simulink model "Full_Motor_Sim"  (R2020b)
settings: Solver=VariableStepAuto  StartTime=0.0  StopTime=1  RelTol=1e-3
libraries: fl_lib x26, ee_lib x20, nesl_utility x19, simulink x12
(part 1 of 2)
settings Model: Creator=1  LastModifiedBy=1
settings SimscapeCC: SimscapeLogType=all  SimscapeLogOpenViewer=on  SimscapeLogName=simlog_ee_igbt  SimscapeLogLimitData=off

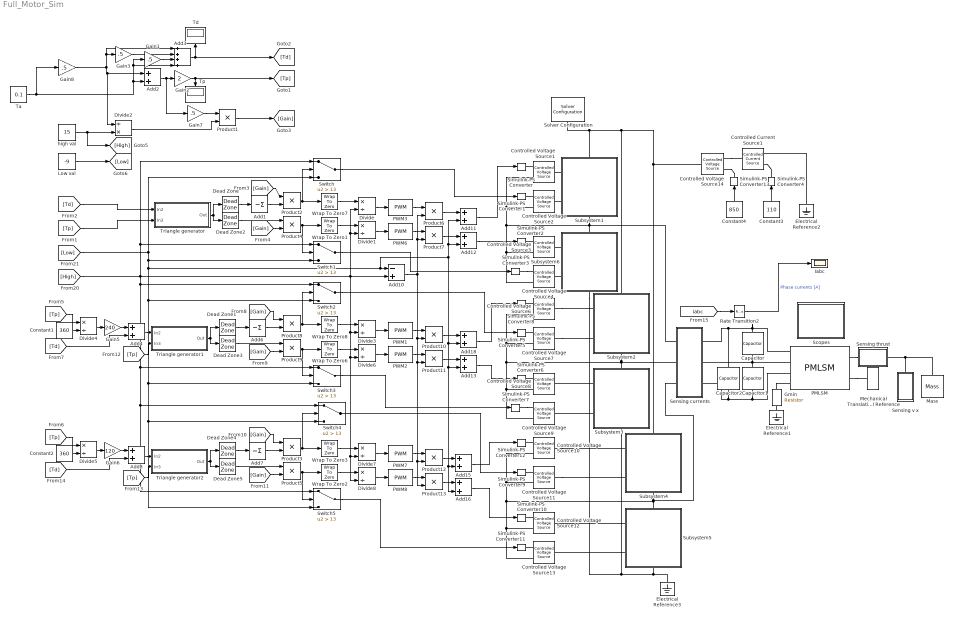
== system Full_Motor_Sim ==
  Add1 : Sum  Inputs=-
  Add10 : Sum  Inputs=-+
  Add{2,4,8,11..13,15..16,18} (9 alike) : Sum
  Add3 : Sum  Inputs=++++
  Add6 : Sum  Inputs=-
  Add7 : Sum  Inputs=-
  Capacitor : fl_lib/Electrical/Electrical Elements/Capacitor  c=1e-4 F  r=0 Ohm  g=0 1/Ohm  i_specify=off  i_priority=None  i=0 A  i_nominal_specify=off  i_nominal_unit=A  i_nominal_value=1  v_specify=off  v_priority=None  v=0 V  v_nominal_specify=off  v_nominal_unit=V  v_nominal_value=1  vc_specify=off  vc_priority=High  vc=0 V  vc_nominal_specify=off  vc_nominal_unit=V  vc_nominal_value=1
  Capacitor1 : fl_lib/Electrical/Electrical Elements/Capacitor  c=1e-4 F  r=0 Ohm  g=0 1/Ohm  i_specify=off  i_priority=None  i=0 A  i_nominal_specify=off  i_nominal_unit=A  i_nominal_value=1  v_specify=off  v_priority=None  v=0 V  v_nominal_specify=off  v_nominal_unit=V  v_nominal_value=1  vc_specify=off  vc_priority=High  vc=0 V  vc_nominal_specify=off  vc_nominal_unit=V  vc_nominal_value=1
  Capacitor2 : fl_lib/Electrical/Electrical Elements/Capacitor  c=1e-4 F  r=0 Ohm  g=0 1/Ohm  i_specify=off  i_priority=None  i=0 A  i_nominal_specify=off  i_nominal_unit=A  i_nominal_value=1  v_specify=off  v_priority=None  v=0 V  v_nominal_specify=off  v_nominal_unit=V  v_nominal_value=1  vc_specify=off  vc_priority=High  vc=0 V  vc_nominal_specify=off  vc_nominal_unit=V  vc_nominal_value=1
  Constant1 : Constant  Value=360
  Constant2 : Constant  Value=360
  Constant3 : Constant  Value=110
  Constant4 : Constant  Value=850
  Controlled Current Source1 : fl_lib/Electrical/Electrical Sources/Controlled Current Source
  Controlled Voltage Source{1..4,6..14} (13 alike) : fl_lib/Electrical/Electrical Sources/Controlled Voltage Source
  Dead Zone : DeadZone  LowerValue=0  UpperValue=18  SaturateOnIntegerOverflow=on
  Dead Zone1 : DeadZone  LowerValue=0  UpperValue=18  SaturateOnIntegerOverflow=on
  Dead Zone2 : DeadZone  LowerValue=-18  UpperValue=0  SaturateOnIntegerOverflow=on
  Dead Zone3 : DeadZone  LowerValue=-18  UpperValue=0  SaturateOnIntegerOverflow=on
  Dead Zone4 : DeadZone  LowerValue=0  UpperValue=18  SaturateOnIntegerOverflow=on
  Dead Zone5 : DeadZone  LowerValue=-18  UpperValue=0  SaturateOnIntegerOverflow=on
  Divide{,1,3..8} (8 alike) : Product  Inputs=*/
  Divide2 : Product  Inputs=/*
  Electrical Reference1 : fl_lib/Electrical/Electrical Elements/Electrical Reference
      settings: SourceProductName=Foundation Library
  Electrical Reference2 : fl_lib/Electrical/Electrical Elements/Electrical Reference
      settings: SourceProductName=Foundation Library
  Electrical Reference3 : fl_lib/Electrical/Electrical Elements/Electrical Reference
      settings: SourceProductName=Foundation Library
  Gain{1,3,7..8} (4 alike) : Gain  Gain=.5
  Gain2 : Gain  Gain=2
  Gain5 : Gain  Gain=240
  Gain6 : Gain  Gain=120
  Gmin : fl_lib/Electrical/Electrical Elements/Resistor  R=1e9 Ohm  i_specify=off  i_priority=High  i=0 A  i_nominal_specify=off  i_nominal_unit=A  i_nominal_value=1  v_specify=off  v_priority=High  v=0 V  v_nominal_specify=off  v_nominal_unit=V  v_nominal_value=1
      settings: SourceProductName=Foundation Library
  Iabc : Scope
  "Low val " : Constant  Value=-9
  Mass : fl_lib/Mechanical/Translational Elements/Mass  mass=7.5 kg  num_ports=foundation.enum.numPorts2.one  v_specify=off  v_priority=High  v=0 m/s  v_nominal_specify=off  v_nominal_unit=m/s  v_nominal_value=1  f_specify=off  f_priority=None  f=0 N  f_nominal_specify=off  f_nominal_unit=N  f_nominal_value=1
      settings: SourceProductName=Foundation Library
  Mechanical Translational Reference : fl_lib/Mechanical/Translational Elements/Mechanical Translational Reference
      settings: SourceProductName=Foundation Library
  PMLSM : ee_lib/Electromechanical/Permanent Magnet/PMLSM  winding_type=ee.enum.statorconnection.wye  machine_param=ee.enum.pmsm.parameterization.constant  polarPitch=16 mm  pmflux_param=ee.enum.pmfluxlin.backemfconstant  pm_flux_linkage=PM Wb  force_constant=0.18 N/A  back_emf_constant=15.75 s*V/m  stator_param=ee.enum.statorparam.LsLmMs  Ld=Ld H  Lq=Lq H  idVec=[-200, 0, 200] A  iqVec=[-200, 0, 200] A  LdMatrix=0.00019 * ones(3, 3) H  LqMatrix=0.00025 * ones(3, 3) H  PmMatrix=0.03 * ones(3, 3) Wb  kfMatrix=0.18 * ones(3, 3) N/A  keMatrix=0.18 * ones(3, 3) s*V/m  L0=L0 H  Ls=0.00077 H  Lm=-0.000077 H  Ms=0.0000385 H  Rs=0.254 Ohm  zero_sequence=ee.enum.park.zerosequence.include  M=7.5 kg  lam=0 N/(m/s)  axes_param=ee.enum.rotorangle.qaxis  i_d_specify=off  i_d_priority=None  i_d=0 A  i_d_nominal_specify=off  i_d_nominal_unit=A  i_d_nominal_value=1  i_q_specify=off  i_q_priority=None  i_q=0 A  i_q_nominal_specify=off  i_q_nominal_unit=A  i_q_nominal_value=1  force_specify=off  force_priority=None  force=0 N  force_nominal_specify=off  force_nominal_unit=N  force_nominal_value=1  linear_velocity_specify=off  linear_velocity_priority=High  linear_velocity=0 m/s  linear_velocity_nominal_specify=off  linear_velocity_nominal_unit=m/s  linear_velocity_nominal_value=1  linear_position_specify=off  linear_position_priority=High  linear_position=0 m  linear_position_nominal_specify=off  linear_position_nominal_unit=m  linear_position_nominal_value=1
      settings: SourceProductName=Electrical  InternalSimscapePortConfiguration="{\"Bottom\":[],\"Left\":[{\"id\":\"a\",\"label\":\"a\",\"type\":\"foundation.electrical.electrical\"},{\"id\":\"b\",\"label\":\"b\",\"type\":\"foundation.electrical.electrical\"},{\"id\":\"c\",\"label\":\"c\",\"type\":\"foundation.electrical.electrical\"},{\"id\":\"n\",\"label\":\"n\",\"type\":\"foundation.electrical.electrical\"}],\"Right\":[{\"id\":\"R\",\"label\":\"R\",\"type\":\"foundation.mechanical.translational.translational\"},{\"id\":\"C\",\"label\":\"C\",\"type\":\"foundation.mechanical.translational.translational\"}],\"Top\":[]}"
  PWM{1..3,6..8} (6 alike) : simulink/Discontinuities/PWM  DisableCoverage=on  Period=0.005  DisallowZeroDutyCycle=off  RunAtFixedTimeIntervals=off  SampleTime=0.1
  Product{1..13} (13 alike) : Product
  Rate Transition2 : RateTransition  OutPortSampleTime=Tsc
  Scopes : Subsystem
  Sensing currents : Subsystem
      mask Display: disp('iabc')
  Sensing thrust : Subsystem
      mask Display: disp('thrust')
  Sensing v x : Subsystem
      mask Display: disp('v,x')
  Simulink-PS Converter{,1..3,5..13} (13 alike) : nesl_utility/Simulink-PS Converter  PhysicalDomain=network_engine_domain  SubClassName=ps_input  LeftPortType=input  RightPortType=output  PseudoPeriodic=off  Frequencies=[]  NoiseDistribution=none  NoiseParameters=[]  Unit=V  AffineConversion=off  FilteringAndDerivatives=provide  SimscapeFilterOrder=1  InputFilterTimeConstant=0.001  UdotUserProvided=0
  Simulink-PS Converter4 : nesl_utility/Simulink-PS Converter  PhysicalDomain=network_engine_domain  SubClassName=ps_input  LeftPortType=input  RightPortType=output  PseudoPeriodic=off  Frequencies=[]  NoiseDistribution=none  NoiseParameters=[]  Unit=A  AffineConversion=off  FilteringAndDerivatives=provide  SimscapeFilterOrder=1  InputFilterTimeConstant=0.001  UdotUserProvided=0
  Solver Configuration : nesl_utility/Solver Configuration  PhysicalDomain=network_engine_domain  SubClassName=solver  LeftPortType=input  RightPortType=generic  Tones=[]  Harmonics=[]  SimulateNoise=off  Profile=off  UseLocalSampling=off  EnableSwitchedLinearOptims=on  FrequencyDomain=off  UseCCode=off  RelTol=0.001  AbsTol=1e-06  MinStep=1e-09  ToWorkspace=off  RevertToSquareIcSolve=off  NumHomotopyIterations=100  PhasorMode=off  PhasorModeNumHarmonics=1  DoDC=on  ResidualTolerance=1e-9  UseLocalSolver=on  LocalSolverChoice=NE_BACKWARD_EULER_ADVANCER  LocalSolverSampleTime=5e-6  DoFixedCost=off  MaxNonlinIter=50  MaxModeIter=2  ComputeImpulses=on  ImpulseIterations=2  LinearAlgebra=auto  EquationFormulation=NE_TIME_EF  DelaysMemoryBudget=2048  AutomaticFiltering=on  FilteringTimeConstant=0.001  PartitionStorageMethod=AS_NEEDED  PartitionMemoryBudget=1024  PartitionMethod=FAST
      settings: SourceProductName=Utilities
  Subsystem1 : Subsystem
      settings: PortSchema="{\"entries\":[{\"content\":{\"sides\":[{\"content\":{\"connectorIds\":[\"LConn1\",\"LConn2\"]},\"type\":\"ConnectorPlacement.EquallySpacedRectSide\",\"uuid\":\"28828598-fa48-4158-b9b9-1a24f22427e6\"},{\"content\":{\"connectorIds\":[],\"side\":\"RIGHT\"},\"type\":\"ConnectorPlacement.EquallySpacedRectSide\",\"uuid\":\"019dad23-614b-4455-8161-a0bd3c38edbe\"},{\"content\":{\"connectorIds\":[\"LConn3\"],\"side\":\"TOP\"},\"type\":\"ConnectorPlacement.EquallySpacedRectSide\",\"uuid\":\"f897a393-49e1-4ff6-9d33-08f3737db00c\"},{\"content\":{\"connectorIds\":[\"RConn1\"],\"side\":\"BOTTOM\"},\"type\":\"ConnectorPlacement.EquallySpacedRectSide\",\"uuid\":\"06fb1490-05e8-4341-9bc6-3d6044d20c9b\"},{\"content\":{\"connectorIds\":[],\"side\":\"HIDDEN\"},\"type\":\"ConnectorPlacement.EquallySpacedRectSide\",\"uuid\":\"25a0668a-edb0-4932-9c2b-b08682b30f2f\"}]},\"type\":\"ConnectorPlacement.EquallySpacedConnector\",\"uuid\":\"66e20cb6-4eb1-4857-9faa-51f0324dd946\"}],\"packageUris\":[\"http://schema.mathworks.com/mf0/Connector/R2020b\"],\"version\":\"1.0\"}"
  Subsystem2 : Subsystem
      settings: PortSchema="{\"entries\":[{\"content\":{\"sides\":[{\"content\":{\"connectorIds\":[\"LConn1\",\"LConn2\"]},\"type\":\"ConnectorPlacement.EquallySpacedRectSide\",\"uuid\":\"28828598-fa48-4158-b9b9-1a24f22427e6\"},{\"content\":{\"connectorIds\":[],\"side\":\"RIGHT\"},\"type\":\"ConnectorPlacement.EquallySpacedRectSide\",\"uuid\":\"019dad23-614b-4455-8161-a0bd3c38edbe\"},{\"content\":{\"connectorIds\":[\"LConn3\"],\"side\":\"TOP\"},\"type\":\"ConnectorPlacement.EquallySpacedRectSide\",\"uuid\":\"f897a393-49e1-4ff6-9d33-08f3737db00c\"},{\"content\":{\"connectorIds\":[\"RConn1\"],\"side\":\"BOTTOM\"},\"type\":\"ConnectorPlacement.EquallySpacedRectSide\",\"uuid\":\"06fb1490-05e8-4341-9bc6-3d6044d20c9b\"},{\"content\":{\"connectorIds\":[],\"side\":\"HIDDEN\"},\"type\":\"ConnectorPlacement.EquallySpacedRectSide\",\"uuid\":\"25a0668a-edb0-4932-9c2b-b08682b30f2f\"}]},\"type\":\"ConnectorPlacement.EquallySpacedConnector\",\"uuid\":\"66e20cb6-4eb1-4857-9faa-51f0324dd946\"}],\"packageUris\":[\"http://schema.mathworks.com/mf0/Connector/R2020b\"],\"version\":\"1.0\"}"
  Subsystem3 : Subsystem
      settings: PortSchema="{\"entries\":[{\"content\":{\"sides\":[{\"content\":{\"connectorIds\":[\"LConn1\",\"LConn2\"]},\"type\":\"ConnectorPlacement.EquallySpacedRectSide\",\"uuid\":\"28828598-fa48-4158-b9b9-1a24f22427e6\"},{\"content\":{\"connectorIds\":[],\"side\":\"RIGHT\"},\"type\":\"ConnectorPlacement.EquallySpacedRectSide\",\"uuid\":\"019dad23-614b-4455-8161-a0bd3c38edbe\"},{\"content\":{\"connectorIds\":[\"LConn3\"],\"side\":\"TOP\"},\"type\":\"ConnectorPlacement.EquallySpacedRectSide\",\"uuid\":\"f897a393-49e1-4ff6-9d33-08f3737db00c\"},{\"content\":{\"connectorIds\":[\"RConn1\"],\"side\":\"BOTTOM\"},\"type\":\"ConnectorPlacement.EquallySpacedRectSide\",\"uuid\":\"e6a9b99e-6cfc-43a0-9f1a-1d6bb159a832\"},{\"content\":{\"connectorIds\":[],\"side\":\"HIDDEN\"},\"type\":\"ConnectorPlacement.EquallySpacedRectSide\",\"uuid\":\"25a0668a-edb0-4932-9c2b-b08682b30f2f\"}]},\"type\":\"ConnectorPlacement.EquallySpacedConnector\",\"uuid\":\"66e20cb6-4eb1-4857-9faa-51f0324dd946\"}],\"packageUris\":[\"http://schema.mathworks.com/mf0/Connector/R2020b\"],\"version\":\"1.0\"}"
  Subsystem4 : Subsystem
      settings: PortSchema="{\"entries\":[{\"content\":{\"sides\":[{\"content\":{\"connectorIds\":[\"LConn1\",\"LConn2\"]},\"type\":\"ConnectorPlacement.EquallySpacedRectSide\",\"uuid\":\"28828598-fa48-4158-b9b9-1a24f22427e6\"},{\"content\":{\"connectorIds\":[],\"side\":\"RIGHT\"},\"type\":\"ConnectorPlacement.EquallySpacedRectSide\",\"uuid\":\"019dad23-614b-4455-8161-a0bd3c38edbe\"},{\"content\":{\"connectorIds\":[\"LConn3\"],\"side\":\"TOP\"},\"type\":\"ConnectorPlacement.EquallySpacedRectSide\",\"uuid\":\"f897a393-49e1-4ff6-9d33-08f3737db00c\"},{\"content\":{\"connectorIds\":[\"RConn1\"],\"side\":\"BOTTOM\"},\"type\":\"ConnectorPlacement.EquallySpacedRectSide\",\"uuid\":\"06fb1490-05e8-4341-9bc6-3d6044d20c9b\"},{\"content\":{\"connectorIds\":[],\"side\":\"HIDDEN\"},\"type\":\"ConnectorPlacement.EquallySpacedRectSide\",\"uuid\":\"25a0668a-edb0-4932-9c2b-b08682b30f2f\"}]},\"type\":\"ConnectorPlacement.EquallySpacedConnector\",\"uuid\":\"66e20cb6-4eb1-4857-9faa-51f0324dd946\"}],\"packageUris\":[\"http://schema.mathworks.com/mf0/Connector/R2020b\"],\"version\":\"1.0\"}"
  Subsystem5 : Subsystem
      settings: PortSchema="{\"entries\":[{\"content\":{\"sides\":[{\"content\":{\"connectorIds\":[\"LConn1\",\"LConn2\"]},\"type\":\"ConnectorPlacement.EquallySpacedRectSide\",\"uuid\":\"28828598-fa48-4158-b9b9-1a24f22427e6\"},{\"content\":{\"connectorIds\":[],\"side\":\"RIGHT\"},\"type\":\"ConnectorPlacement.EquallySpacedRectSide\",\"uuid\":\"019dad23-614b-4455-8161-a0bd3c38edbe\"},{\"content\":{\"connectorIds\":[\"LConn3\"],\"side\":\"TOP\"},\"type\":\"ConnectorPlacement.EquallySpacedRectSide\",\"uuid\":\"f897a393-49e1-4ff6-9d33-08f3737db00c\"},{\"content\":{\"connectorIds\":[\"RConn1\"],\"side\":\"BOTTOM\"},\"type\":\"ConnectorPlacement.EquallySpacedRectSide\",\"uuid\":\"e6a9b99e-6cfc-43a0-9f1a-1d6bb159a832\"},{\"content\":{\"connectorIds\":[],\"side\":\"HIDDEN\"},\"type\":\"ConnectorPlacement.EquallySpacedRectSide\",\"uuid\":\"25a0668a-edb0-4932-9c2b-b08682b30f2f\"}]},\"type\":\"ConnectorPlacement.EquallySpacedConnector\",\"uuid\":\"66e20cb6-4eb1-4857-9faa-51f0324dd946\"}],\"packageUris\":[\"http://schema.mathworks.com/mf0/Connector/R2020b\"],\"version\":\"1.0\"}"
  Subsystem6 : Subsystem
      settings: PortSchema="{\"entries\":[{\"content\":{\"sides\":[{\"content\":{\"connectorIds\":[\"LConn1\",\"LConn2\"]},\"type\":\"ConnectorPlacement.EquallySpacedRectSide\",\"uuid\":\"28828598-fa48-4158-b9b9-1a24f22427e6\"},{\"content\":{\"connectorIds\":[],\"side\":\"RIGHT\"},\"type\":\"ConnectorPlacement.EquallySpacedRectSide\",\"uuid\":\"019dad23-614b-4455-8161-a0bd3c38edbe\"},{\"content\":{\"connectorIds\":[\"LConn3\"],\"side\":\"TOP\"},\"type\":\"ConnectorPlacement.EquallySpacedRectSide\",\"uuid\":\"f897a393-49e1-4ff6-9d33-08f3737db00c\"},{\"content\":{\"connectorIds\":[\"RConn1\"],\"side\":\"BOTTOM\"},\"type\":\"ConnectorPlacement.EquallySpacedRectSide\",\"uuid\":\"e6a9b99e-6cfc-43a0-9f1a-1d6bb159a832\"},{\"content\":{\"connectorIds\":[],\"side\":\"HIDDEN\"},\"type\":\"ConnectorPlacement.EquallySpacedRectSide\",\"uuid\":\"25a0668a-edb0-4932-9c2b-b08682b30f2f\"}]},\"type\":\"ConnectorPlacement.EquallySpacedConnector\",\"uuid\":\"66e20cb6-4eb1-4857-9faa-51f0324dd946\"}],\"packageUris\":[\"http://schema.mathworks.com/mf0/Connector/R2020b\"],\"version\":\"1.0\"}"
  Switch{,1..5} (6 alike) : Switch  Criteria=u2 > Threshold  Threshold=13
  Ta : Constant  Value=0.1
  Td : Display
  Tp : Display
  Triangle generator : Subsystem
  Triangle generator1 : Subsystem
  Triangle generator2 : Subsystem
  Wrap To Zero{1..3,6..8} (6 alike) : simulink/Discontinuities/Wrap To Zero  Threshold=15
      settings: SourceProductBaseCode=SL
  "high val " : Constant  Value=15
  wires:
  Gain2/1 -> [Tp], Tp/1
  [Tp] -> Triangle generator/2(In3)
  Ta/1 -> Gain8/1, Gain1/1, Add3/4, Add2/2
  Add2/1 -> Gain7/1, Gain2/1
  Gain8/1 -> Add2/1, Divide2/1, Gain3/1, Add3/1
  Dead Zone/1 -> Add1/1
  Triangle generator/1(Out) -> Dead Zone/1, Dead Zone2/1
  Gain1/1 -> Add3/3
  [Td] -> Triangle generator/1(In2)
  Add1/1 -> Product2/2
  [Gain] -> Product2/1
  Dead Zone2/1 -> Product4/1
  [Gain] -> Product4/2
  [Tp] -> Divide4/1
  Constant1/1 -> Divide4/2
  Divide4/1 -> Gain5/1
  Divide5/1 -> Gain6/1
  Constant2/1 -> Divide5/2
  [Tp] -> Divide5/1
  Gain5/1 -> Add4/1
  Gain6/1 -> Add8/1
  [Td] -> Add4/2
  [Gain] -> Product9/2
  Dead Zone3/1 -> Product9/1
  [Gain] -> Product8/1
  Add6/1 -> Product8/2
  Triangle generator1/1(Out) -> Dead Zone3/1, Dead Zone1/1
  Dead Zone1/1 -> Add6/1
  Add4/1 -> Triangle generator1/1(In2)
  Dead Zone4/1 -> Add7/1
  Triangle generator2/1(Out) -> Dead Zone4/1, Dead Zone5/1
  Add7/1 -> Product3/2
  [Gain] -> Product3/1
  Dead Zone5/1 -> Product5/1
  [Gain] -> Product5/2
  Add8/1 -> Triangle generator2/1(In2)
  [Tp] -> Triangle generator2/2(In3)
  [Tp] -> Triangle generator1/2(In3)
  "high val "/1 -> [High], Divide2/2
  Gain7/1 -> Product1/1
  Divide2/1 -> Product1/2
  Product1/1 -> [Gain]
  Product2/1 -> Switch/2, Wrap To Zero7/1
  Product4/1 -> Switch1/2, Wrap To Zero1/1
  [Td] -> Add8/2
  Product8/1 -> Wrap To Zero8/1, Switch2/2
  Product3/1 -> Switch4/2, Wrap To Zero3/1
  Product5/1 -> Switch5/2, Wrap To Zero2/1
  Product9/1 -> Wrap To Zero6/1, Switch3/2
  [Low] -> Switch2/3, Switch3/3, Switch4/3, Switch5/3, Add18/2, Add13/2, Add16/2, Add15/2, Add11/2, Add12/2, Add10/1, Switch1/3, Switch/3
  Switch5/1 -> Simulink-PS Converter11/1
  Switch4/1 -> Simulink-PS Converter9/1
  Switch2/1 -> Simulink-PS Converter5/1
  Switch3/1 -> Simulink-PS Converter7/1
  Switch1/1 -> Simulink-PS Converter3/1
  Wrap To Zero7/1 -> Divide/1
  Wrap To Zero1/1 -> Divide1/1
  Divide/1 -> PWM3/1
  Divide1/1 -> PWM6/1
  PWM3/1 -> Product6/1
  PWM6/1 -> Product7/1
  Add3/1 -> Td/1, [Td]
  PWM2/1 -> Product11/1
  PWM1/1 -> Product10/1
  Divide6/1 -> PWM2/1
  Divide3/1 -> PWM1/1
  Wrap To Zero6/1 -> Divide6/1
  Wrap To Zero8/1 -> Divide3/1
  Wrap To Zero3/1 -> Divide7/1
  Wrap To Zero2/1 -> Divide8/1
  [High] -> Switch3/1, Switch4/1, Switch5/1, Switch2/1, Switch1/1, Switch/1, Add10/2, Divide3/2, Divide6/2, Divide8/2, Divide7/2, Divide/2, Divide1/2
  Divide7/1 -> PWM7/1
  Divide8/1 -> PWM8/1
  PWM7/1 -> Product12/1
  PWM8/1 -> Product13/1
  Switch/1 -> Simulink-PS Converter1/1
  Add10/1 -> Product7/2, Product6/2, Product12/2, Product13/2, Product11/2, Product10/2
  "Low val "/1 -> [Low]
  Product6/1 -> Add11/1
  Product7/1 -> Add12/1
  Product11/1 -> Add13/1
  Product10/1 -> Add18/1
  Product13/1 -> Add16/1
  Product12/1 -> Add15/1
  Add11/1 -> Simulink-PS Converter/1
  Add12/1 -> Simulink-PS Converter2/1
  Add18/1 -> Simulink-PS Converter8/1
  Add13/1 -> Simulink-PS Converter6/1
  Add15/1 -> Simulink-PS Converter12/1
  Add16/1 -> Simulink-PS Converter10/1
  Constant3/1 -> Simulink-PS Converter4/1
  Gain3/1 -> Add3/2
  Constant4/1 -> Simulink-PS Converter13/1
  [iabc] -> Rate Transition2/1
  Rate Transition2/1 -> Iabc/1  "Phase currents [A]"
  connections:
  Controlled Voltage Source3/RConn2 -- Sensing currents/LConn1 -- Subsystem6/LConn3 -- Subsystem1/RConn1 -- Controlled Voltage Source2/RConn2 -- Controlled Voltage Source1/RConn2 -- Controlled Voltage Source4/RConn2
  Simulink-PS Converter/RConn1 -- Controlled Voltage Source1/RConn1
  Simulink-PS Converter1/RConn1 -- Controlled Voltage Source2/RConn1
  Simulink-PS Converter2/RConn1 -- Controlled Voltage Source3/RConn1
  Simulink-PS Converter3/RConn1 -- Controlled Voltage Source4/RConn1
  Subsystem1/LConn1 -- Controlled Voltage Source1/LConn1
  Subsystem1/LConn2 -- Controlled Voltage Source2/LConn1
  Subsystem6/LConn1 -- Controlled Voltage Source3/LConn1
  Subsystem6/LConn2 -- Controlled Voltage Source4/LConn1
  Controlled Voltage Source7/RConn2 -- Controlled Voltage Source8/RConn2 -- Controlled Voltage Source9/RConn2 -- Subsystem2/RConn1 -- Subsystem3/LConn3 -- Sensing currents/LConn2 -- Controlled Voltage Source6/RConn2
  Subsystem3/LConn1 -- Controlled Voltage Source8/LConn1
  Simulink-PS Converter7/RConn1 -- Controlled Voltage Source9/RConn1
  Capacitor/RConn1 -- PMLSM/LConn2 -- Capacitor1/LConn1 -- Sensing currents/RConn2
  Simulink-PS Converter6/RConn1 -- Controlled Voltage Source8/RConn1
  Simulink-PS Converter5/RConn1 -- Controlled Voltage Source7/RConn1
  Controlled Voltage Source7/LConn1 -- Subsystem2/LConn2
  Controlled Voltage Source6/LConn1 -- Subsystem2/LConn1
  Subsystem3/LConn2 -- Controlled Voltage Source9/LConn1
  Simulink-PS Converter8/RConn1 -- Controlled Voltage Source6/RConn1
  Subsystem4/RConn1 -- Sensing currents/LConn3 -- Subsystem5/LConn3 -- Controlled Voltage Source13/RConn2 -- Controlled Voltage Source12/RConn2 -- Controlled Voltage Source11/RConn2 -- Controlled Voltage Source10/RConn2
  Simulink-PS Converter12/RConn1 -- Controlled Voltage Source10/RConn1
  Subsystem5/LConn2 -- Controlled Voltage Source13/LConn1
  Controlled Voltage Source10/LConn1 -- Subsystem4/LConn1
  Simulink-PS Converter10/RConn1 -- Controlled Voltage Source12/RConn1
  Capacitor1/RConn1 -- PMLSM/LConn3 -- Capacitor2/RConn1 -- Sensing currents/RConn3
  Simulink-PS Converter11/RConn1 -- Controlled Voltage Source13/RConn1
  Subsystem5/LConn1 -- Controlled Voltage Source12/LConn1
  Simulink-PS Converter9/RConn1 -- Controlled Voltage Source11/RConn1
  Controlled Voltage Source11/LConn1 -- Subsystem4/LConn2
  Simulink-PS Converter4/RConn1 -- Controlled Current Source1/RConn1
  Subsystem4/LConn3 -- Controlled Voltage Source14/LConn1 -- Subsystem2/LConn3 -- Subsystem1/LConn3 -- Solver Configuration/RConn1
  Subsystem5/RConn1 -- Electrical Reference3/LConn1 -- Subsystem6/RConn1 -- Subsystem3/RConn1
  Electrical Reference2/LConn1 -- Controlled Current Source1/RConn2
  Controlled Voltage Source14/RConn2 -- Controlled Current Source1/LConn1
  Controlled Voltage Source14/RConn1 -- Simulink-PS Converter13/RConn1
  Sensing thrust/RConn1 -- Mass/LConn1 -- Sensing v x/LConn1
  Electrical Reference1/LConn1 -- Gmin/LConn1
  Capacitor/LConn1 -- PMLSM/LConn1 -- Capacitor2/LConn1 -- Sensing currents/RConn1
  PMLSM/RConn1 -- Sensing thrust/LConn1
  PMLSM/RConn2 -- Mechanical Translational Reference/LConn1
  PMLSM/LConn4 -- Gmin/RConn1

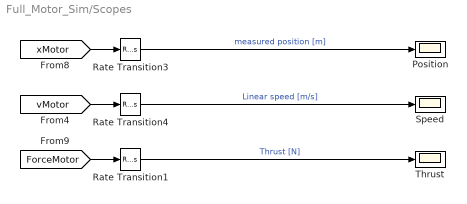
== system Full_Motor_Sim/Scopes ==
  Position : Scope
  Rate Transition1 : RateTransition  OutPortSampleTime=Tsc
  Rate Transition3 : RateTransition  OutPortSampleTime=Tsc
  Rate Transition4 : RateTransition  OutPortSampleTime=Tsc
  Speed : Scope
  Thrust : Scope
  wires:
  Rate Transition4/1 -> Speed/1  "Linear speed [m/s]"
  Rate Transition3/1 -> Position/1  "measured position [m]"
  [xMotor] -> Rate Transition3/1
  Rate Transition1/1 -> Thrust/1  "Thrust [N]"
  [ForceMotor] -> Rate Transition1/1
  [vMotor] -> Rate Transition4/1

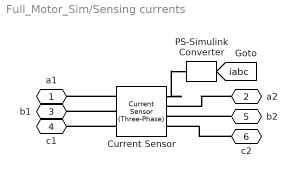
== system Full_Motor_Sim/Sensing currents ==
  Current Sensor : ee_lib/Sensors & Transducers/Current Sensor (Three-Phase)
      settings: SourceProductName=Electrical  InternalSimscapePortConfiguration="{\"Bottom\":[],\"Left\":[{\"id\":\"a1\",\"label\":\"a1\",\"type\":\"foundation.electrical.electrical\"},{\"id\":\"b1\",\"label\":\"b1\",\"type\":\"foundation.electrical.electrical\"},{\"id\":\"c1\",\"label\":\"c1\",\"type\":\"foundation.electrical.electrical\"}],\"Right\":[{\"id\":\"I_output\",\"label\":\"I\",\"type\":\"output\"},{\"id\":\"a2\",\"label\":\"a2\",\"type\":\"foundation.electrical.electrical\"},{\"id\":\"b2\",\"label\":\"b2\",\"type\":\"foundation.electrical.electrical\"},{\"id\":\"c2\",\"label\":\"c2\",\"type\":\"foundation.electrical.electrical\"}],\"Top\":[]}"
  PS-Simulink Converter : nesl_utility/PS-Simulink Converter  PhysicalDomain=network_engine_domain  SubClassName=ps_output  LeftPortType=input  RightPortType=output  PseudoPeriodic=off  Frequencies=[]  Unit=A  AffineConversion=off
      settings: SourceProductName=Utilities
  a1 : PMIOPort  Side=Left
  a2 : PMIOPort  Port=2  Side=Right
  b1 : PMIOPort  Port=3  Side=Left
  c1 : PMIOPort  Port=4  Side=Left
  b2 : PMIOPort  Port=5  Side=Right
  c2 : PMIOPort  Port=6  Side=Right
  tag scope: iabc=global
  wires:
  PS-Simulink Converter/1 -> [iabc]
  connections:
  Current Sensor/LConn1 -- a1/RConn1
  a2/RConn1 -- Current Sensor/RConn2
  Current Sensor/RConn1 -- PS-Simulink Converter/LConn1
  Current Sensor/LConn2 -- b1/RConn1
  Current Sensor/LConn3 -- c1/RConn1
  b2/RConn1 -- Current Sensor/RConn3
  c2/RConn1 -- Current Sensor/RConn4

== system Full_Motor_Sim/Sensing thrust ==
  Ideal Force Sensor : fl_lib/Mechanical/Mechanical Sensors/Ideal Force Sensor
      settings: SourceProductName=Foundation Library
  PS-Simulink Converter2 : nesl_utility/PS-Simulink Converter  PhysicalDomain=network_engine_domain  SubClassName=ps_output  LeftPortType=input  RightPortType=output  PseudoPeriodic=off  Frequencies=[]  Unit=N  AffineConversion=off
      settings: SourceProductName=Utilities
  C : PMIOPort  Side=Right
  R : PMIOPort  Port=2  Side=Left
  tag scope: ForceMotor=global
  wires:
  PS-Simulink Converter2/1 -> [ForceMotor]
  connections:
  Ideal Force Sensor/RConn1 -- C/RConn1
  Ideal Force Sensor/RConn2 -- PS-Simulink Converter2/LConn1
  Ideal Force Sensor/LConn1 -- R/RConn1

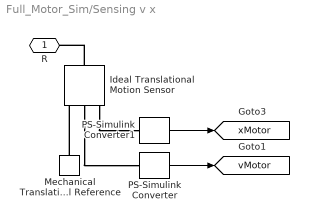
== system Full_Motor_Sim/Sensing v x ==
  Ideal Translational Motion Sensor : fl_lib/Mechanical/Mechanical Sensors/Ideal Translational Motion Sensor  offset=0 m
      settings: SourceProductName=Foundation Library
  Mechanical Translational Reference : fl_lib/Mechanical/Translational Elements/Mechanical Translational Reference
      settings: SourceProductName=Foundation Library
  PS-Simulink Converter : nesl_utility/PS-Simulink Converter  PhysicalDomain=network_engine_domain  SubClassName=ps_output  LeftPortType=input  RightPortType=output  PseudoPeriodic=off  Frequencies=[]  Unit=m/s  AffineConversion=off
      settings: SourceProductName=Utilities
  PS-Simulink Converter1 : nesl_utility/PS-Simulink Converter  PhysicalDomain=network_engine_domain  SubClassName=ps_output  LeftPortType=input  RightPortType=output  PseudoPeriodic=off  Frequencies=[]  Unit=m  AffineConversion=off
      settings: SourceProductName=Utilities
  R : PMIOPort  Side=Left
  tag scope: vMotor=global, xMotor=global
  wires:
  PS-Simulink Converter1/1 -> [xMotor]
  PS-Simulink Converter/1 -> [vMotor]
  connections:
  Ideal Translational Motion Sensor/RConn2 -- PS-Simulink Converter/LConn1
  Ideal Translational Motion Sensor/LConn1 -- R/RConn1
  Ideal Translational Motion Sensor/RConn3 -- PS-Simulink Converter1/LConn1
  Mechanical Translational Reference/LConn1 -- Ideal Translational Motion Sensor/RConn1

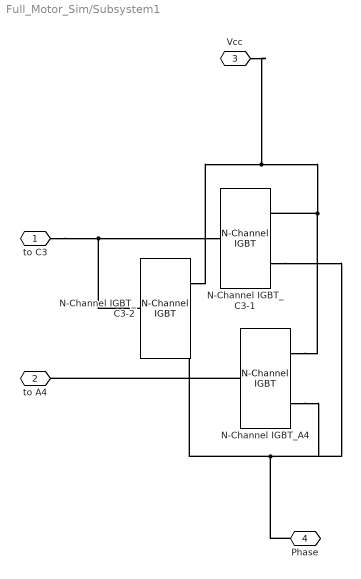
== system Full_Motor_Sim/Subsystem1 ==
  N-Channel IGBT_A4 : ee_lib/Semiconductors & Converters/N-Channel IGBT  model_type=1  Ices=25 uA  Vces=1200 V  Vth=5 V  Vce_sat=1.4 V  Ice_sat=110 A  Vge_sat=15 V  ec=1.3  Tmeas=25 degC  Vge_vec=[ -2 6 7 8 10 12 15 20 ] V  Vce_vec=[ -1 0 0.5 1 1.5 2 2.5 3 3.5 4 ] V  T_vec=[25, 125] degC  Ic_mat=[ -1.015e-5 1.35e-8 4.7135e-4 5.092e-4 5.105e-4 5.117500000000001e-4 5.1299e-4 5.1423e-4 5.1548e-4 5.1672e-4; -9.986899999999999e-6 1.35e-8 4.7135e-4 5.092e-4 5.105e-4 5.117500000000001e-4 5.1299e-4 5.1423e-4 5.1548e-4 5.1672e-4; -9.955e-6 1.35e-8 0.0065225 3.3324 48.154 93.661 105.52 105.72 105.93 106.14; -9.955e-6 1.35e-8 0.0065235 3.5783 70.264 166.33 252.4 317.67 353.38 357.39; -9.955e-6 1.35e-8 0.006524 3.7206 89.17100000000001 228.09 371.63 511.02 642.6900000000001 764.04; -9.9549e-6 1.35e-8 0.0065242 3.7716 97.79300000000001 256.21 424.27 592.92 759.2 921.52; -9.9549e-6 1.35e-8 0.0065243 3.8067 104.52 278.11 464.6 654.37 844.5700000000001 1.0339e+3; -9.9549e-6 1.35e-8 0.0065244 3.8324 109.92 295.67 496.54 702.28 909.96 1.1183e+3 ] A  Ic_mat_3D=zeros(8, 10, 2) A  C_param=3  C_GE=23.7 nF  C_GC=2.7 nF  C_CE=0 nF  C_ies=9.85 nF  C_res=218 pF  C_oes=580 pF  C_GE_vec=[ 25 31 26.5 24.9 25 24.9 24.6 24.7 24.8 ] nF  C_GC_vec=[ 55 9 5.5 3.1 2.5 2.1 1.9 1.8 1.7 ] nF  C_CE_vec=[ 5 11 6.5 4.9 3.5 2.7 2.1 1.7 1.4 ] nF  C_ies_vec=[70 62 60 60 60 60 60 60 60 ] nF  C_res_vec=[ 12 0.46 0.32 0.28 0.24 0.22 0.2 0.19 0.16 ] nF  C_oes_vec=[ 31 0.73 0.515 0.44 0.38 0.34 0.31 0.29 0.28 ] nF  C_Vce_vec=[ 0 5 10 15 20 25 30 35 40 ] V  charge_linearity_param=1  C_OX=20 nF  V_C_OX=-5 V  TF=0 ns  VAF=350 V  RC=0.0001 Ohm  RE=0.0045 Ohm  RG=1 Ohm  BF=100  T_param=2  Ices_T2=620 uA  EG=0.0001 eV  Vce_sat_T2=1.6 V  Tmeas2=150 degC  XTI=1  BEX=-0.6  RG_alpha=1 1/K  Tdevice=150 degC  Tdevice_3D=25 degC  thermal_network_parameterization=ee.enum.thermalNetworkTopology.cauer  Rth=[0, 10] K/W  Rth_Foster=[4, 6] K/W  thermal_mass_parameterization=ee.enum.thermalNetwork.timeconstant  thermal_mass=[0, 1] J/K  thermal_mass_Foster=[1.5, 3] J/K  thermal_time_constant=[0, 10] s  thermal_time_constant_Foster=[6, 18] s  thermal_mass_initial_temperatures=[25, 25] degC  Ic_vec1=[0, 10, 50, 100, 200, 400, 600] A  Vce_vec1=[0, 1.1, 1.3, 1.45, 1.75, 2.25, 2.7] V  Rmiller=0.1 Ohm  Goff=1e-5 1/Ohm  t_on=0.07 us  t_rise=0.7 us  t_off=0.2 us  t_fall=0.5 us  v_meas=300 V  Tj_vec1=[298.15, 398.15] K  Vce_mat1=[0, 1.1, 1.3, 1.45, 1.75, 2.25, 2.7; 0, 1, 1.15, 1.35, 1.7, 2.35, 3] V  E_turn_on_mat1=[0, .2, 1, 2, 4, 8, 15; 0, .3, 1.3, 2.5, 5, 11, 18] * 1e-3 J  E_turn_off_mat1=[0, .3, 1.5, 3, 6, 15, 25; 0, .7, 3.3, 6.5, 13, 25, 35] * 1e-3 J
      settings: SourceProductBaseCode=PS  InternalSimscapePortConfiguration="{\"Bottom\":[],\"Left\":[{\"id\":\"G\",\"label\":\"\",\"type\":\"foundation.electrical.electrical\"}],\"Right\":[{\"id\":\"C\",\"label\":\"\",\"type\":\"foundation.electrical.electrical\"},{\"id\":\"E\",\"label\":\"\",\"type\":\"foundation.electrical.electrical\"}],\"Top\":[]}"
  N-Channel IGBT_C3-1 : ee_lib/Semiconductors & Converters/N-Channel IGBT  model_type=1  Ices=25 uA  Vces=1200 V  Vth=5 V  Vce_sat=2.25 V  Ice_sat=40 A  Vge_sat=7 V  ec=1.5  Tmeas=25 degC  Vge_vec=[ -2 6 7 8 10 12 15 20 ] V  Vce_vec=[ -1 0 0.5 1 1.5 2 2.5 3 3.5 4 ] V  T_vec=[25, 125] degC  Ic_mat=[ -1.015e-5 1.35e-8 4.7135e-4 5.092e-4 5.105e-4 5.117500000000001e-4 5.1299e-4 5.1423e-4 5.1548e-4 5.1672e-4; -9.986899999999999e-6 1.35e-8 4.7135e-4 5.092e-4 5.105e-4 5.117500000000001e-4 5.1299e-4 5.1423e-4 5.1548e-4 5.1672e-4; -9.955e-6 1.35e-8 0.0065225 3.3324 48.154 93.661 105.52 105.72 105.93 106.14; -9.955e-6 1.35e-8 0.0065235 3.5783 70.264 166.33 252.4 317.67 353.38 357.39; -9.955e-6 1.35e-8 0.006524 3.7206 89.17100000000001 228.09 371.63 511.02 642.6900000000001 764.04; -9.9549e-6 1.35e-8 0.0065242 3.7716 97.79300000000001 256.21 424.27 592.92 759.2 921.52; -9.9549e-6 1.35e-8 0.0065243 3.8067 104.52 278.11 464.6 654.37 844.5700000000001 1.0339e+3; -9.9549e-6 1.35e-8 0.0065244 3.8324 109.92 295.67 496.54 702.28 909.96 1.1183e+3 ] A  Ic_mat_3D=zeros(8, 10, 2) A  C_param=3  C_GE=23.7 nF  C_GC=2.7 nF  C_CE=0 nF  C_ies=9.85 nF  C_res=218 pF  C_oes=580 pF  C_GE_vec=[ 25 31 26.5 24.9 25 24.9 24.6 24.7 24.8 ] nF  C_GC_vec=[ 55 9 5.5 3.1 2.5 2.1 1.9 1.8 1.7 ] nF  C_CE_vec=[ 5 11 6.5 4.9 3.5 2.7 2.1 1.7 1.4 ] nF  C_ies_vec=[ 18 13 12 11 10 10 10 10 10 ] nF  C_res_vec=[ 6 2.7 1.9 1.3 0.36 0.22 0.19 0.17 0.16 ] nF  C_oes_vec=[ 8.5 4 3 2 0.8 0.6 0.5 0.48 0.43 ] nF  C_Vce_vec=[ 0 5 10 15 20 25 30 35 40 ] V  charge_linearity_param=1  C_OX=20 nF  V_C_OX=-5 V  TF=0 ns  VAF=10 V  RC=0.005 Ohm  RE=0.009 Ohm  RG=1 kOhm  BF=100  T_param=2  Ices_T2=1.5 mA  EG=0.0001 eV  Vce_sat_T2=2.45 V  Tmeas2=150 degC  XTI=1  BEX=-1  RG_alpha=1 1/K  Tdevice=150 degC  Tdevice_3D=25 degC  thermal_network_parameterization=ee.enum.thermalNetworkTopology.cauer  Rth=[0, 10] K/W  Rth_Foster=[4, 6] K/W  thermal_mass_parameterization=ee.enum.thermalNetwork.timeconstant  thermal_mass=[0, 1] J/K  thermal_mass_Foster=[1.5, 3] J/K  thermal_time_constant=[0, 10] s  thermal_time_constant_Foster=[6, 18] s  thermal_mass_initial_temperatures=[25, 25] degC  Ic_vec1=[0, 10, 50, 100, 200, 400, 600] A  Vce_vec1=[0, 1.1, 1.3, 1.45, 1.75, 2.25, 2.7] V  Rmiller=0.1 Ohm  Goff=1e-5 1/Ohm  t_on=0.07 us  t_rise=0.7 us  t_off=0.2 us  t_fall=0.5 us  v_meas=300 V  Tj_vec1=[298.15, 398.15] K  Vce_mat1=[0, 1.1, 1.3, 1.45, 1.75, 2.25, 2.7; 0, 1, 1.15, 1.35, 1.7, 2.35, 3] V  E_turn_on_mat1=[0, .2, 1, 2, 4, 8, 15; 0, .3, 1.3, 2.5, 5, 11, 18] * 1e-3 J  E_turn_off_mat1=[0, .3, 1.5, 3, 6, 15, 25; 0, .7, 3.3, 6.5, 13, 25, 35] * 1e-3 J
      settings: SourceProductName=Electrical  InternalSimscapePortConfiguration="{\"Bottom\":[],\"Left\":[{\"id\":\"G\",\"label\":\"\",\"type\":\"foundation.electrical.electrical\"}],\"Right\":[{\"id\":\"C\",\"label\":\"\",\"type\":\"foundation.electrical.electrical\"},{\"id\":\"E\",\"label\":\"\",\"type\":\"foundation.electrical.electrical\"}],\"Top\":[]}"
  N-Channel IGBT_C3-2 : ee_lib/Semiconductors & Converters/N-Channel IGBT  model_type=1  Ices=25 uA  Vces=1200 V  Vth=5 V  Vce_sat=2.25 V  Ice_sat=40 A  Vge_sat=7 V  ec=1.5  Tmeas=25 degC  Vge_vec=[ -2 6 7 8 10 12 15 20 ] V  Vce_vec=[ -1 0 0.5 1 1.5 2 2.5 3 3.5 4 ] V  T_vec=[25, 125] degC  Ic_mat=[ -1.015e-5 1.35e-8 4.7135e-4 5.092e-4 5.105e-4 5.117500000000001e-4 5.1299e-4 5.1423e-4 5.1548e-4 5.1672e-4; -9.986899999999999e-6 1.35e-8 4.7135e-4 5.092e-4 5.105e-4 5.117500000000001e-4 5.1299e-4 5.1423e-4 5.1548e-4 5.1672e-4; -9.955e-6 1.35e-8 0.0065225 3.3324 48.154 93.661 105.52 105.72 105.93 106.14; -9.955e-6 1.35e-8 0.0065235 3.5783 70.264 166.33 252.4 317.67 353.38 357.39; -9.955e-6 1.35e-8 0.006524 3.7206 89.17100000000001 228.09 371.63 511.02 642.6900000000001 764.04; -9.9549e-6 1.35e-8 0.0065242 3.7716 97.79300000000001 256.21 424.27 592.92 759.2 921.52; -9.9549e-6 1.35e-8 0.0065243 3.8067 104.52 278.11 464.6 654.37 844.5700000000001 1.0339e+3; -9.9549e-6 1.35e-8 0.0065244 3.8324 109.92 295.67 496.54 702.28 909.96 1.1183e+3 ] A  Ic_mat_3D=zeros(8, 10, 2) A  C_param=3  C_GE=23.7 nF  C_GC=2.7 nF  C_CE=0 nF  C_ies=9.85 nF  C_res=218 pF  C_oes=580 pF  C_GE_vec=[ 25 31 26.5 24.9 25 24.9 24.6 24.7 24.8 ] nF  C_GC_vec=[ 55 9 5.5 3.1 2.5 2.1 1.9 1.8 1.7 ] nF  C_CE_vec=[ 5 11 6.5 4.9 3.5 2.7 2.1 1.7 1.4 ] nF  C_ies_vec=[ 18 13 12 11 10 10 10 10 10 ] nF  C_res_vec=[ 6 2.7 1.9 1.3 0.36 0.22 0.19 0.17 0.16 ] nF  C_oes_vec=[ 8.5 4 3 2 0.8 0.6 0.5 0.48 0.43 ] nF  C_Vce_vec=[ 0 5 10 15 20 25 30 35 40 ] V  charge_linearity_param=1  C_OX=20 nF  V_C_OX=-5 V  TF=0 ns  VAF=10 V  RC=0.005 Ohm  RE=0.009 Ohm  RG=1 kOhm  BF=100  T_param=2  Ices_T2=1.5 mA  EG=0.0001 eV  Vce_sat_T2=2.45 V  Tmeas2=150 degC  XTI=1  BEX=-1  RG_alpha=1 1/K  Tdevice=150 degC  Tdevice_3D=25 degC  thermal_network_parameterization=ee.enum.thermalNetworkTopology.cauer  Rth=[0, 10] K/W  Rth_Foster=[4, 6] K/W  thermal_mass_parameterization=ee.enum.thermalNetwork.timeconstant  thermal_mass=[0, 1] J/K  thermal_mass_Foster=[1.5, 3] J/K  thermal_time_constant=[0, 10] s  thermal_time_constant_Foster=[6, 18] s  thermal_mass_initial_temperatures=[25, 25] degC  Ic_vec1=[0, 10, 50, 100, 200, 400, 600] A  Vce_vec1=[0, 1.1, 1.3, 1.45, 1.75, 2.25, 2.7] V  Rmiller=0.1 Ohm  Goff=1e-5 1/Ohm  t_on=0.07 us  t_rise=0.7 us  t_off=0.2 us  t_fall=0.5 us  v_meas=300 V  Tj_vec1=[298.15, 398.15] K  Vce_mat1=[0, 1.1, 1.3, 1.45, 1.75, 2.25, 2.7; 0, 1, 1.15, 1.35, 1.7, 2.35, 3] V  E_turn_on_mat1=[0, .2, 1, 2, 4, 8, 15; 0, .3, 1.3, 2.5, 5, 11, 18] * 1e-3 J  E_turn_off_mat1=[0, .3, 1.5, 3, 6, 15, 25; 0, .7, 3.3, 6.5, 13, 25, 35] * 1e-3 J
      settings: SourceProductName=Electrical  InternalSimscapePortConfiguration="{\"Bottom\":[],\"Left\":[{\"id\":\"G\",\"label\":\"\",\"type\":\"foundation.electrical.electrical\"}],\"Right\":[{\"id\":\"C\",\"label\":\"\",\"type\":\"foundation.electrical.electrical\"},{\"id\":\"E\",\"label\":\"\",\"type\":\"foundation.electrical.electrical\"}],\"Top\":[]}"
  to C3 : PMIOPort  Side=Left
  to A4 : PMIOPort  Port=2  Side=Left
  Vcc : PMIOPort  Port=3  Side=Left
  Phase : PMIOPort  Port=4  Side=Right
  connections:
  N-Channel IGBT_A4/LConn1 -- to A4/RConn1
  N-Channel IGBT_C3-2/LConn1 -- to C3/RConn1 -- N-Channel IGBT_C3-1/LConn1
  Phase/RConn1 -- N-Channel IGBT_A4/RConn2 -- N-Channel IGBT_C3-1/RConn2 -- N-Channel IGBT_C3-2/RConn2
  Vcc/RConn1 -- N-Channel IGBT_C3-2/RConn1 -- N-Channel IGBT_A4/RConn1 -- N-Channel IGBT_C3-1/RConn1

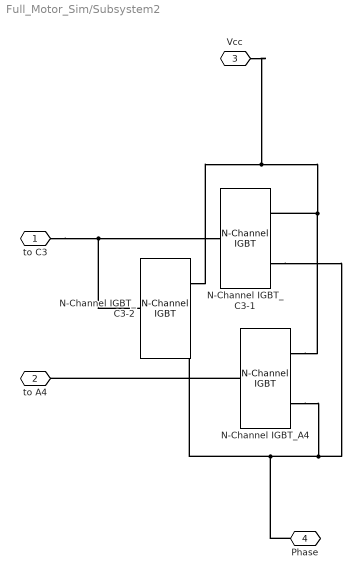
== system Full_Motor_Sim/Subsystem2 ==
  N-Channel IGBT_A4 : ee_lib/Semiconductors & Converters/N-Channel IGBT  model_type=1  Ices=25 uA  Vces=1200 V  Vth=5 V  Vce_sat=1.4 V  Ice_sat=110 A  Vge_sat=15 V  ec=1.3  Tmeas=25 degC  Vge_vec=[ -2 6 7 8 10 12 15 20 ] V  Vce_vec=[ -1 0 0.5 1 1.5 2 2.5 3 3.5 4 ] V  T_vec=[25, 125] degC  Ic_mat=[ -1.015e-5 1.35e-8 4.7135e-4 5.092e-4 5.105e-4 5.117500000000001e-4 5.1299e-4 5.1423e-4 5.1548e-4 5.1672e-4; -9.986899999999999e-6 1.35e-8 4.7135e-4 5.092e-4 5.105e-4 5.117500000000001e-4 5.1299e-4 5.1423e-4 5.1548e-4 5.1672e-4; -9.955e-6 1.35e-8 0.0065225 3.3324 48.154 93.661 105.52 105.72 105.93 106.14; -9.955e-6 1.35e-8 0.0065235 3.5783 70.264 166.33 252.4 317.67 353.38 357.39; -9.955e-6 1.35e-8 0.006524 3.7206 89.17100000000001 228.09 371.63 511.02 642.6900000000001 764.04; -9.9549e-6 1.35e-8 0.0065242 3.7716 97.79300000000001 256.21 424.27 592.92 759.2 921.52; -9.9549e-6 1.35e-8 0.0065243 3.8067 104.52 278.11 464.6 654.37 844.5700000000001 1.0339e+3; -9.9549e-6 1.35e-8 0.0065244 3.8324 109.92 295.67 496.54 702.28 909.96 1.1183e+3 ] A  Ic_mat_3D=zeros(8, 10, 2) A  C_param=3  C_GE=23.7 nF  C_GC=2.7 nF  C_CE=0 nF  C_ies=9.85 nF  C_res=218 pF  C_oes=580 pF  C_GE_vec=[ 25 31 26.5 24.9 25 24.9 24.6 24.7 24.8 ] nF  C_GC_vec=[ 55 9 5.5 3.1 2.5 2.1 1.9 1.8 1.7 ] nF  C_CE_vec=[ 5 11 6.5 4.9 3.5 2.7 2.1 1.7 1.4 ] nF  C_ies_vec=[70 62 60 60 60 60 60 60 60 ] nF  C_res_vec=[ 12 0.46 0.32 0.28 0.24 0.22 0.2 0.19 0.16 ] nF  C_oes_vec=[ 31 0.73 0.515 0.44 0.38 0.34 0.31 0.29 0.28 ] nF  C_Vce_vec=[ 0 5 10 15 20 25 30 35 40 ] V  charge_linearity_param=1  C_OX=20 nF  V_C_OX=-5 V  TF=0 ns  VAF=350 V  RC=0.0001 Ohm  RE=0.0045 Ohm  RG=1 Ohm  BF=100  T_param=2  Ices_T2=620 uA  EG=0.0001 eV  Vce_sat_T2=1.6 V  Tmeas2=150 degC  XTI=1  BEX=-0.6  RG_alpha=1 1/K  Tdevice=150 degC  Tdevice_3D=25 degC  thermal_network_parameterization=ee.enum.thermalNetworkTopology.cauer  Rth=[0, 10] K/W  Rth_Foster=[4, 6] K/W  thermal_mass_parameterization=ee.enum.thermalNetwork.timeconstant  thermal_mass=[0, 1] J/K  thermal_mass_Foster=[1.5, 3] J/K  thermal_time_constant=[0, 10] s  thermal_time_constant_Foster=[6, 18] s  thermal_mass_initial_temperatures=[25, 25] degC  Ic_vec1=[0, 10, 50, 100, 200, 400, 600] A  Vce_vec1=[0, 1.1, 1.3, 1.45, 1.75, 2.25, 2.7] V  Rmiller=0.1 Ohm  Goff=1e-5 1/Ohm  t_on=0.07 us  t_rise=0.7 us  t_off=0.2 us  t_fall=0.5 us  v_meas=300 V  Tj_vec1=[298.15, 398.15] K  Vce_mat1=[0, 1.1, 1.3, 1.45, 1.75, 2.25, 2.7; 0, 1, 1.15, 1.35, 1.7, 2.35, 3] V  E_turn_on_mat1=[0, .2, 1, 2, 4, 8, 15; 0, .3, 1.3, 2.5, 5, 11, 18] * 1e-3 J  E_turn_off_mat1=[0, .3, 1.5, 3, 6, 15, 25; 0, .7, 3.3, 6.5, 13, 25, 35] * 1e-3 J
      settings: SourceProductBaseCode=PS  InternalSimscapePortConfiguration="{\"Bottom\":[],\"Left\":[{\"id\":\"G\",\"label\":\"\",\"type\":\"foundation.electrical.electrical\"}],\"Right\":[{\"id\":\"C\",\"label\":\"\",\"type\":\"foundation.electrical.electrical\"},{\"id\":\"E\",\"label\":\"\",\"type\":\"foundation.electrical.electrical\"}],\"Top\":[]}"
  N-Channel IGBT_C3-1 : ee_lib/Semiconductors & Converters/N-Channel IGBT  model_type=1  Ices=25 uA  Vces=1200 V  Vth=5 V  Vce_sat=2.25 V  Ice_sat=40 A  Vge_sat=7 V  ec=1.5  Tmeas=25 degC  Vge_vec=[ -2 6 7 8 10 12 15 20 ] V  Vce_vec=[ -1 0 0.5 1 1.5 2 2.5 3 3.5 4 ] V  T_vec=[25, 125] degC  Ic_mat=[ -1.015e-5 1.35e-8 4.7135e-4 5.092e-4 5.105e-4 5.117500000000001e-4 5.1299e-4 5.1423e-4 5.1548e-4 5.1672e-4; -9.986899999999999e-6 1.35e-8 4.7135e-4 5.092e-4 5.105e-4 5.117500000000001e-4 5.1299e-4 5.1423e-4 5.1548e-4 5.1672e-4; -9.955e-6 1.35e-8 0.0065225 3.3324 48.154 93.661 105.52 105.72 105.93 106.14; -9.955e-6 1.35e-8 0.0065235 3.5783 70.264 166.33 252.4 317.67 353.38 357.39; -9.955e-6 1.35e-8 0.006524 3.7206 89.17100000000001 228.09 371.63 511.02 642.6900000000001 764.04; -9.9549e-6 1.35e-8 0.0065242 3.7716 97.79300000000001 256.21 424.27 592.92 759.2 921.52; -9.9549e-6 1.35e-8 0.0065243 3.8067 104.52 278.11 464.6 654.37 844.5700000000001 1.0339e+3; -9.9549e-6 1.35e-8 0.0065244 3.8324 109.92 295.67 496.54 702.28 909.96 1.1183e+3 ] A  Ic_mat_3D=zeros(8, 10, 2) A  C_param=3  C_GE=23.7 nF  C_GC=2.7 nF  C_CE=0 nF  C_ies=9.85 nF  C_res=218 pF  C_oes=580 pF  C_GE_vec=[ 25 31 26.5 24.9 25 24.9 24.6 24.7 24.8 ] nF  C_GC_vec=[ 55 9 5.5 3.1 2.5 2.1 1.9 1.8 1.7 ] nF  C_CE_vec=[ 5 11 6.5 4.9 3.5 2.7 2.1 1.7 1.4 ] nF  C_ies_vec=[ 18 13 12 11 10 10 10 10 10 ] nF  C_res_vec=[ 6 2.7 1.9 1.3 0.36 0.22 0.19 0.17 0.16 ] nF  C_oes_vec=[ 8.5 4 3 2 0.8 0.6 0.5 0.48 0.43 ] nF  C_Vce_vec=[ 0 5 10 15 20 25 30 35 40 ] V  charge_linearity_param=1  C_OX=20 nF  V_C_OX=-5 V  TF=0 ns  VAF=10 V  RC=0.005 Ohm  RE=0.009 Ohm  RG=1 kOhm  BF=100  T_param=2  Ices_T2=1.5 mA  EG=0.0001 eV  Vce_sat_T2=2.45 V  Tmeas2=150 degC  XTI=1  BEX=-1  RG_alpha=1 1/K  Tdevice=150 degC  Tdevice_3D=25 degC  thermal_network_parameterization=ee.enum.thermalNetworkTopology.cauer  Rth=[0, 10] K/W  Rth_Foster=[4, 6] K/W  thermal_mass_parameterization=ee.enum.thermalNetwork.timeconstant  thermal_mass=[0, 1] J/K  thermal_mass_Foster=[1.5, 3] J/K  thermal_time_constant=[0, 10] s  thermal_time_constant_Foster=[6, 18] s  thermal_mass_initial_temperatures=[25, 25] degC  Ic_vec1=[0, 10, 50, 100, 200, 400, 600] A  Vce_vec1=[0, 1.1, 1.3, 1.45, 1.75, 2.25, 2.7] V  Rmiller=0.1 Ohm  Goff=1e-5 1/Ohm  t_on=0.07 us  t_rise=0.7 us  t_off=0.2 us  t_fall=0.5 us  v_meas=300 V  Tj_vec1=[298.15, 398.15] K  Vce_mat1=[0, 1.1, 1.3, 1.45, 1.75, 2.25, 2.7; 0, 1, 1.15, 1.35, 1.7, 2.35, 3] V  E_turn_on_mat1=[0, .2, 1, 2, 4, 8, 15; 0, .3, 1.3, 2.5, 5, 11, 18] * 1e-3 J  E_turn_off_mat1=[0, .3, 1.5, 3, 6, 15, 25; 0, .7, 3.3, 6.5, 13, 25, 35] * 1e-3 J
      settings: SourceProductName=Electrical  InternalSimscapePortConfiguration="{\"Bottom\":[],\"Left\":[{\"id\":\"G\",\"label\":\"\",\"type\":\"foundation.electrical.electrical\"}],\"Right\":[{\"id\":\"C\",\"label\":\"\",\"type\":\"foundation.electrical.electrical\"},{\"id\":\"E\",\"label\":\"\",\"type\":\"foundation.electrical.electrical\"}],\"Top\":[]}"
  N-Channel IGBT_C3-2 : ee_lib/Semiconductors & Converters/N-Channel IGBT  model_type=1  Ices=25 uA  Vces=1200 V  Vth=5 V  Vce_sat=2.25 V  Ice_sat=40 A  Vge_sat=7 V  ec=1.5  Tmeas=25 degC  Vge_vec=[ -2 6 7 8 10 12 15 20 ] V  Vce_vec=[ -1 0 0.5 1 1.5 2 2.5 3 3.5 4 ] V  T_vec=[25, 125] degC  Ic_mat=[ -1.015e-5 1.35e-8 4.7135e-4 5.092e-4 5.105e-4 5.117500000000001e-4 5.1299e-4 5.1423e-4 5.1548e-4 5.1672e-4; -9.986899999999999e-6 1.35e-8 4.7135e-4 5.092e-4 5.105e-4 5.117500000000001e-4 5.1299e-4 5.1423e-4 5.1548e-4 5.1672e-4; -9.955e-6 1.35e-8 0.0065225 3.3324 48.154 93.661 105.52 105.72 105.93 106.14; -9.955e-6 1.35e-8 0.0065235 3.5783 70.264 166.33 252.4 317.67 353.38 357.39; -9.955e-6 1.35e-8 0.006524 3.7206 89.17100000000001 228.09 371.63 511.02 642.6900000000001 764.04; -9.9549e-6 1.35e-8 0.0065242 3.7716 97.79300000000001 256.21 424.27 592.92 759.2 921.52; -9.9549e-6 1.35e-8 0.0065243 3.8067 104.52 278.11 464.6 654.37 844.5700000000001 1.0339e+3; -9.9549e-6 1.35e-8 0.0065244 3.8324 109.92 295.67 496.54 702.28 909.96 1.1183e+3 ] A  Ic_mat_3D=zeros(8, 10, 2) A  C_param=3  C_GE=23.7 nF  C_GC=2.7 nF  C_CE=0 nF  C_ies=9.85 nF  C_res=218 pF  C_oes=580 pF  C_GE_vec=[ 25 31 26.5 24.9 25 24.9 24.6 24.7 24.8 ] nF  C_GC_vec=[ 55 9 5.5 3.1 2.5 2.1 1.9 1.8 1.7 ] nF  C_CE_vec=[ 5 11 6.5 4.9 3.5 2.7 2.1 1.7 1.4 ] nF  C_ies_vec=[ 18 13 12 11 10 10 10 10 10 ] nF  C_res_vec=[ 6 2.7 1.9 1.3 0.36 0.22 0.19 0.17 0.16 ] nF  C_oes_vec=[ 8.5 4 3 2 0.8 0.6 0.5 0.48 0.43 ] nF  C_Vce_vec=[ 0 5 10 15 20 25 30 35 40 ] V  charge_linearity_param=1  C_OX=20 nF  V_C_OX=-5 V  TF=0 ns  VAF=10 V  RC=0.005 Ohm  RE=0.009 Ohm  RG=1 kOhm  BF=100  T_param=2  Ices_T2=1.5 mA  EG=0.0001 eV  Vce_sat_T2=2.45 V  Tmeas2=150 degC  XTI=1  BEX=-1  RG_alpha=1 1/K  Tdevice=150 degC  Tdevice_3D=25 degC  thermal_network_parameterization=ee.enum.thermalNetworkTopology.cauer  Rth=[0, 10] K/W  Rth_Foster=[4, 6] K/W  thermal_mass_parameterization=ee.enum.thermalNetwork.timeconstant  thermal_mass=[0, 1] J/K  thermal_mass_Foster=[1.5, 3] J/K  thermal_time_constant=[0, 10] s  thermal_time_constant_Foster=[6, 18] s  thermal_mass_initial_temperatures=[25, 25] degC  Ic_vec1=[0, 10, 50, 100, 200, 400, 600] A  Vce_vec1=[0, 1.1, 1.3, 1.45, 1.75, 2.25, 2.7] V  Rmiller=0.1 Ohm  Goff=1e-5 1/Ohm  t_on=0.07 us  t_rise=0.7 us  t_off=0.2 us  t_fall=0.5 us  v_meas=300 V  Tj_vec1=[298.15, 398.15] K  Vce_mat1=[0, 1.1, 1.3, 1.45, 1.75, 2.25, 2.7; 0, 1, 1.15, 1.35, 1.7, 2.35, 3] V  E_turn_on_mat1=[0, .2, 1, 2, 4, 8, 15; 0, .3, 1.3, 2.5, 5, 11, 18] * 1e-3 J  E_turn_off_mat1=[0, .3, 1.5, 3, 6, 15, 25; 0, .7, 3.3, 6.5, 13, 25, 35] * 1e-3 J
      settings: SourceProductName=Electrical  InternalSimscapePortConfiguration="{\"Bottom\":[],\"Left\":[{\"id\":\"G\",\"label\":\"\",\"type\":\"foundation.electrical.electrical\"}],\"Right\":[{\"id\":\"C\",\"label\":\"\",\"type\":\"foundation.electrical.electrical\"},{\"id\":\"E\",\"label\":\"\",\"type\":\"foundation.electrical.electrical\"}],\"Top\":[]}"
  to C3 : PMIOPort  Side=Left
  to A4 : PMIOPort  Port=2  Side=Left
  Vcc : PMIOPort  Port=3  Side=Left
  Phase : PMIOPort  Port=4  Side=Right
  connections:
  N-Channel IGBT_A4/LConn1 -- to A4/RConn1
  N-Channel IGBT_C3-2/LConn1 -- to C3/RConn1 -- N-Channel IGBT_C3-1/LConn1
  Phase/RConn1 -- N-Channel IGBT_A4/RConn2 -- N-Channel IGBT_C3-1/RConn2 -- N-Channel IGBT_C3-2/RConn2
  Vcc/RConn1 -- N-Channel IGBT_C3-2/RConn1 -- N-Channel IGBT_A4/RConn1 -- N-Channel IGBT_C3-1/RConn1
